simulink model "AIE_RTL_cosim_black_box"  (R2023a)
settings: Solver=VariableStepAuto  StartTime=0.0  StopTime=4000  RelTol=1e-3
PreLoadFcn:
  | xmcCheckSlxPath(bdroot);
  | input = readcomplexdata('./sw/input.h');
  | 
  | % ii of the HDL black box design is 19. Hence we are running
  | % the HDL desgin at 20 times faster than
  | % the input sample time.
  | 
  | sample_time = 0.5/20
InitFcn:
  | xlEvaluateHDLBlocks('AIE_RTL_cosim_black_box')
undefined symbols (not defined in the file): c, S, vsva2197, xcvc1902
libraries: hdlBasic x4, aieUtilities x2, aieBasic x2, hdlUtilities x2, simulink x1, dspsrcs4 x1, vmcUtilities x1
settings Model: Creator=abehbood  LastModifiedBy=robg
settings SolverCC: AlgebraicLoopSolver=TrustRegion
settings DebuggingCC: UnconnectedInputMsg=warning  UnconnectedOutputMsg=warning  UnconnectedLineMsg=warning
settings ModelReferenceCC: EnableRefExpFcnMdlSchedulingChecks=on
settings SFSimCC: CustomCodeUndefinedFunction=UseInterfaceOnly
settings RTWCC: DLArmComputeVersion=19.05

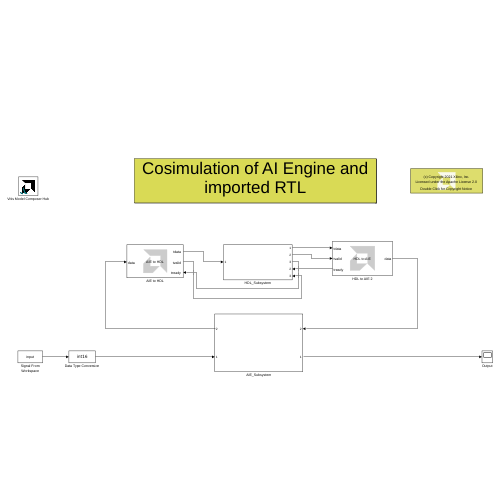
[thumbnail: Simulink's stored preview of the top-level diagram]
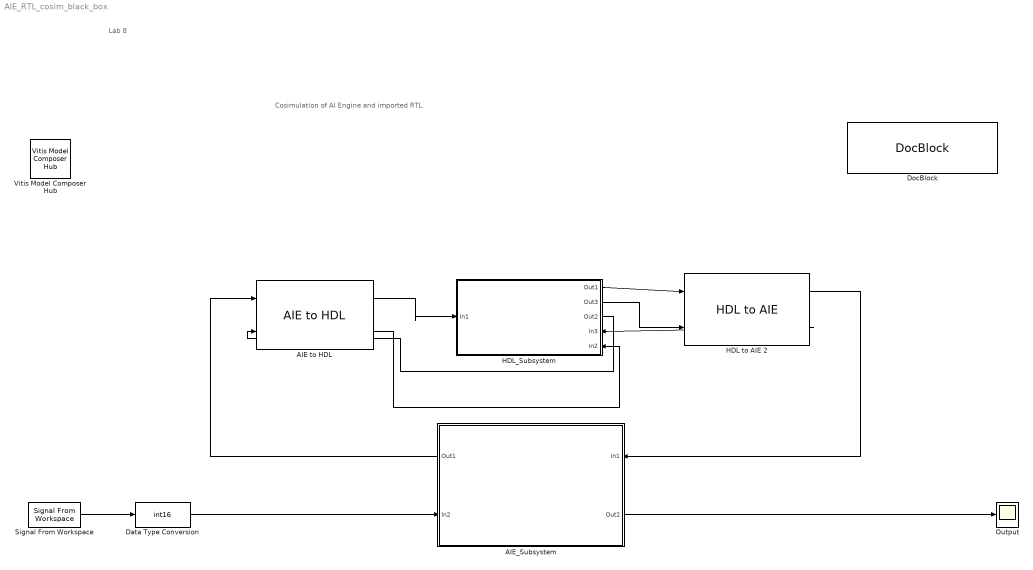
== system AIE_RTL_cosim_black_box ==
  note: Lab 8
  note: Cosimulation of AI Engine and imported RTL
  AIE to HDL : aieUtilities/AIE to HDL  OutDataType=uint32  OutSampleTime=Inherit: Same as tready
  AIE_Subsystem : Subsystem
      settings: PortSchema="{\"entries\":[{\"content\":{\"sides\":[{\"content\":{\"connectorIds\":[\"Out2\",\"In1\"]},\"type\":\"ConnectorPlacement.EquallySpacedRectSide\",\"uuid\":\"898d8c47-e932-4e65-b4ee-22fcab4c971c\"},{\"content\":{\"connectorIds\":[\"In2\",\"Out1\"],\"side\":\"RIGHT\"},\"type\":\"ConnectorPlacement.EquallySpacedRectSide\",\"uuid\":\"af23ae14-2da0-4d61-8b36-3a1d0e7ee3d3\"},{\"content\":{\"connectorIds\":[],\"side\":\"TOP\"},\"type\":\"ConnectorPlacement.EquallySpacedRectSide\",\"uuid\":\"f5229823-660d-4ed4-bac1-26d92dde4203\"}]},\"type\":\"ConnectorPlacement.EquallySpacedConnector\",\"uuid\":\"c8995052-e1b5-42bb-bdd0-b566c20174a5\"}],\"packageUris\":[\"http://schema.mathworks.com/mf0/Connector/19700101\"],\"version\":\"1.0\"}"
  Data Type Conversion : DataTypeConversion  OutDataTypeStr=int16  SaturateOnIntegerOverflow=off  RndMeth=Floor
  DocBlock : simulink/Model-Wide Utilities/DocBlock  DocumentType=Text  mask(DocBlock){}
      content=|
      | ///////////////////////////////////////////////////////////////////////////
      | // Copyright 2021 Xilinx
      | //
      | // Licensed under the Apache License, Version 2.0 (the "License");
      | // you may not use this file except in compliance with the License.
      | // You may obtain a copy of the License at
      | //
      | // http://www.apache.org/licenses/LICENSE-2.0
      | //
      | // Unless required by applicable law or agreed to in writing, software
      | // distributed under the License is distributed on an "AS IS" BASIS,
      | // WITHOUT WARRANTIES OR CONDITIONS OF ANY KIND, either express or implied.
      | // See the License for the specific language governing permissions and
      | // limitations under the License.
      | ///////////////////////////////////////////////////////////////////////////
      mask Display:
      | xmcDrawBlockIcon();
      | disp(['{\fontsize{10pt}(c) Copyright 2021' ' Xilinx, Inc.}\newline \newline '],'texmode','on');
      | disp('{\fontsize{10pt}Licensed under the Apache License 2.0}','texmode','on');
      | disp('\newline \newline \newline{\fontsize{10pt}Double Click for Copyright Notice}','texmode','on');
  HDL to AIE 2 : aieUtilities/HDL to AIE  InDataType=uint32  OutDataType=int16 (c)  OutSampleTime=.5  SamplesPerFrame=256  RateReduceFactor=1  ManuallySpecifyOutSampleTime=on
  HDL_Subsystem : Subsystem
      settings: PortSchema="{\"entries\":[{\"content\":{\"sides\":[{\"content\":{\"connectorIds\":[\"In1\"]},\"type\":\"ConnectorPlacement.EquallySpacedRectSide\",\"uuid\":\"f7d09b9b-9cab-45de-a234-ce17189f1f38\"},{\"content\":{\"connectorIds\":[\"Out1\",\"Out2\",\"Out3\",\"In2\",\"In3\"],\"side\":\"RIGHT\"},\"type\":\"ConnectorPlacement.EquallySpacedRectSide\",\"uuid\":\"963e2550-c982-4a72-83e5-f36d54b36baa\"},{\"content\":{\"connectorIds\":[],\"side\":\"TOP\"},\"type\":\"ConnectorPlacement.EquallySpacedRectSide\",\"uuid\":\"f90a1520-9218-4692-a090-e2089f523264\"}]},\"type\":\"ConnectorPlacement.EquallySpacedConnector\",\"uuid\":\"882f0c8e-c8d0-442e-9388-2de8afbb4cc9\"}],\"packageUris\":[\"http://schema.mathworks.com/mf0/Connector/R2020b\"],\"version\":\"1.0\"}"
  Output : Scope
  Signal From Workspace : dspsrcs4/Signal From Workspace  X=input  Ts=1  nsamps=128  OutputAfterFinalValue=Setting to zero  ignoreOrWarnInputAndFrameLengths=off  OutputFrames=off
  Vitis Model Composer Hub : vmcUtilities/Vitis Model Composer Hub  Tag=genX  CodeGeneration=off  SubsystemName=HDL_Subsystem  CompilationType=HDLCompilation  ExportTypeV2=IP Catalog  StartColumn=1  NumberOfColumns=1  TargetDirectory=./netlist/ip/HDL_Subsystem/src  exportDesign=off  analyzeDesign=on  validateDesignOnHw=off  ExportType=AI Engines  IpVendor=xilinx.com  IpLibrary=hls  IpVersion=1.0  IpHWLanguage=Verilog  AieCompilerOptions={}  AieSimulatorOptions={}  CreateTestbench=on  TestbenchStackSize=10  RunRtlSim=off  RunCSim=off  RunAieSim=off  AieSimTimeout=50000  RunAieSimProfiling=off  LaunchVitisAnalyzer=off  PlotOutput=off  RunX86Sim=off  X86SimTimeout=10  GenHwImage=off  GenLibadfXo=off  GenHwValidationCode=off  PlatformType=Not Specified  HwSystemType=Linux  HwValidationTarget=hw_emu  CommonSwDir=/proj/xbuilds/CustTA/2022.1_2022_0311_0103/internal_platforms/sw/versal/xilinx-versal-common-v2022.1  SdkDirectory=/proj/xsjhdstaff4/abehbood/petalinux/2022.1  ProjDevice=xcvc1902-vsva2197-1LP-e-S  ProjDevicePart=xcvc1902-vsva2197-1LP-e-S  AIEType=AIE  SamplePeriod=-1  ClockFrequency=200  DataPathParallelism=1  xilinxfamily=versalaicore  part=xcvc1902  speed=-1LP-e-S  package=vsva2197  directory=./netlist/ip/HDL_Subsystem/src  testbench=on  incr_netlist=off  synthesis_tool=Vivado  clock_wrapper=Clock Enables  dbl_ovrd=According to Block Masks  dcm_input_clock_period=10  sysclk_period=10  simulink_period=sample_time  eval_field=0  IPInfoJsonString="{\"HDLSubsystem\":{\"SubsystemName\":\"HDL_Subsystem\",\"IPName\":\"HDL_Subsystem\",\"IPLibrary\":\"VMC\",\"IPVendor\":\"User Company\",\"IPVersion\":\"1.0\",\"TargetDirectory\":\"./netlist\",\"SubsystemDir\":\"./netlist/ip/HDL_Subsystem\"},\"SubsystemTag\":\"HDLNode\"}"  LogFileName=''  NThreads=4
  wires:
  Signal From Workspace/1 -> Data Type Conversion/1
  HDL to AIE 2/1 -> AIE_Subsystem/2(In1)
  Data Type Conversion/1 -> AIE_Subsystem/1(In2)
  AIE_Subsystem/2(Out1) -> AIE to HDL/1
  AIE_Subsystem/1(Out2) -> Output/1
  AIE to HDL/1 -> HDL_Subsystem/1(In1)
  HDL to AIE 2/2 -> HDL_Subsystem/2(In3)
  HDL_Subsystem/1(Out1) -> HDL to AIE 2/1
  HDL_Subsystem/2(Out3) -> HDL to AIE 2/2
  HDL_Subsystem/3(Out2) -> AIE to HDL/2
  AIE to HDL/2 -> HDL_Subsystem/3(In2)

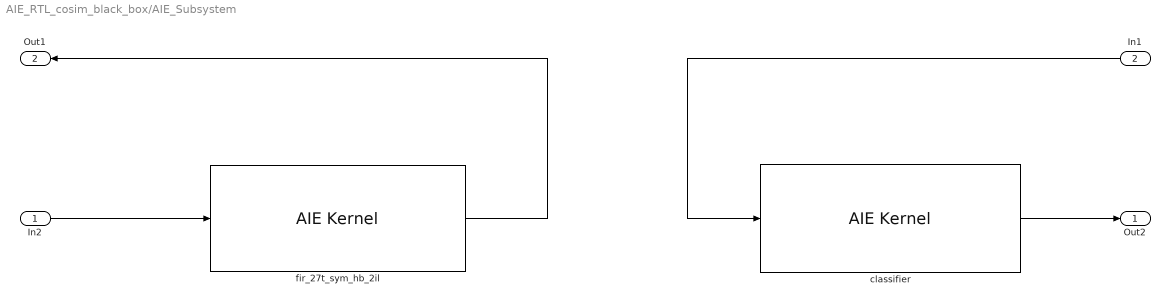
== system AIE_RTL_cosim_black_box/AIE_Subsystem ==
  In2 : Inport
  In1 : Inport  Port=2
  classifier : aieBasic/AIE Kernel  KernelAllAttrs=s[12;12;9;9;19;14;21;23;24;21;12;24;26;26;26;27;28;9;21;23;23;23;24;25;14;19;19;29]@FunctionNameDeclFileNamePortNamesPortTypesPortSerializedTypesPortDirectionsPortWindowSizeEnablesPortWindowMarginEnablesPortSynchronicityEnablesPortSignalSizeEnablesFunctionDeclFunctionTemplateSpecKindFunctionTemplateParamNamesFunctionTemplateParamKindsFunctionTemplateParamTypesFunctionTemplateParamValuesFunctionTemplateParamEnablesClassDeclClassTemplateSpecKindClassTemplateParamNamesClassTemplateParamKindsClassTemplateParamTypesClassTemplateParamValuesClassTemplateParamEnablesClassCtorDeclsClassCtorParamNamesClassCtorParamTypesClassCtorParamSerializedTypes[1 1]@C[28 1]@t10@classifiert19@../../src/kernels.hC[2 1]@t5@inputt6@outputC[2 1]@t21@input_stream_cint16 *t21@output_window_int32 *C[2 1]@t33@{P{Tinput_stream{1{t{Scint16}}}}}t31@{P{Toutput_window{1{t{Bi32}}}}}C[2 1]@t5@inputt6@outputC[2 1]@l0@l1@C[2 1]@l0@l0@C[2 1]@l0@l1@C[2 1]@l0@l0@t74@void classifier(input_stream_cint16 * input, output_window_int32 * output)t4@nonee[0 1]@e[0 1]@e[0 1]@e[0 1]@e[0 1]@nne[0 1]@e[0 1]@e[0 1]@e[0 1]@e[0 1]@e[0 1]@e[0 1]@e[0 1]@e[0 1]@  PortNames={'input'; 'output'}  PortSerializedTypes={'{P{Tinput_stream{1{t{Scint16}}}}}'; '{P{Toutput_window{1{t{Bi32}}}}}'}  PortWindowSizes={0.000000000000000000e+00, 2.560000000000000000e+02}  PortWindowMargins={0.000000000000000000e+00, 0.000000000000000000e+00}  PortSynchronicities={'auto', 'auto'}  PortSignalSizes={0.000000000000000000e+00; 0.000000000000000000e+00}  FunctionTemplateSpecKind=none  FunctionTemplateParamNames={}  FunctionTemplateParamKinds={}  FunctionTemplateParamTypes={}  FunctionTemplateParamValues={}  FunctionIndex=1  FunctionTabVisible=on  FunctionTemplateParamsVisible=off  FunctionDeclTypeOptions=C[1 1]@t74@void classifier(input_stream_cint16 * input, output_window_int32 * output)  FunctionDecl=void classifier(input_stream_cint16 * input, output_window_int32 * output)  FunctionTemplateParams={}  FunctionTemplateParamsEnables={}  PortAttrs={ 'Input', 'input', 'input_stream_cint16 *', '', '', '', ''; 'Output', 'output', 'output_window_int32 *', '256', '', 'auto', '' }  PortAttrsEnables={'off', 'off', 'off', 'off', 'off', 'off', 'off';'off', 'off', 'off', 'on', 'off', 'on', 'off'}  SampleTime=-1  KernelHeaderFile=src/kernels.h  KernelFunction=classifier  KernelSourceFile=src/kernels/classifiers/classify.cc  KernelSearchPaths={}  PreProcOptions={}  blockJsonConstraints=[]
  fir_27t_sym_hb_2il : aieBasic/AIE Kernel  KernelAllAttrs=s[12;12;9;9;19;14;21;23;24;21;12;24;26;26;26;27;28;9;21;23;23;23;24;25;14;19;19;29]@FunctionNameDeclFileNamePortNamesPortTypesPortSerializedTypesPortDirectionsPortWindowSizeEnablesPortWindowMarginEnablesPortSynchronicityEnablesPortSignalSizeEnablesFunctionDeclFunctionTemplateSpecKindFunctionTemplateParamNamesFunctionTemplateParamKindsFunctionTemplateParamTypesFunctionTemplateParamValuesFunctionTemplateParamEnablesClassDeclClassTemplateSpecKindClassTemplateParamNamesClassTemplateParamKindsClassTemplateParamTypesClassTemplateParamValuesClassTemplateParamEnablesClassCtorDeclsClassCtorParamNamesClassCtorParamTypesClassCtorParamSerializedTypes[1 1]@C[28 1]@t17@fir_27t_sym_hb_2it19@../../src/kernels.hC[2 1]@t7@inputcbt8@outputcbC[2 1]@t21@input_window_cint16 *t22@output_window_cint16 *C[2 1]@t33@{P{Tinput_window{1{t{Scint16}}}}}t34@{P{Toutput_window{1{t{Scint16}}}}}C[2 1]@t5@inputt6@outputC[2 1]@l1@l1@C[2 1]@l1@l0@C[2 1]@l1@l1@C[2 1]@l0@l0@t86@void fir_27t_sym_hb_2i(input_window_cint16 * inputcb, output_window_cint16 * outputcb)t4@nonee[0 1]@e[0 1]@e[0 1]@e[0 1]@e[0 1]@nne[0 1]@e[0 1]@e[0 1]@e[0 1]@e[0 1]@e[0 1]@e[0 1]@e[0 1]@e[0 1]@  PortNames={'inputcb'; 'outputcb'}  PortSerializedTypes={'{P{Tinput_window{1{t{Scint16}}}}}'; '{P{Toutput_window{1{t{Scint16}}}}}'}  PortWindowSizes={1.280000000000000000e+02, 2.560000000000000000e+02}  PortWindowMargins={1.600000000000000000e+01, 0.000000000000000000e+00}  PortSynchronicities={'auto', 'auto'}  PortSignalSizes={0.000000000000000000e+00; 0.000000000000000000e+00}  FunctionTemplateSpecKind=none  FunctionTemplateParamNames={}  FunctionTemplateParamKinds={}  FunctionTemplateParamTypes={}  FunctionTemplateParamValues={}  FunctionIndex=1  FunctionTabVisible=on  FunctionTemplateParamsVisible=off  FunctionDeclTypeOptions=C[1 1]@t86@void fir_27t_sym_hb_2i(input_window_cint16 * inputcb, output_window_cint16 * outputcb)  FunctionDecl=void fir_27t_sym_hb_2i(input_window_cint16 * inputcb, output_window_cint16 * outputcb)  FunctionTemplateParams={}  FunctionTemplateParamsEnables={}  PortAttrs={ 'Input','inputcb','input_window_cint16 *','128','16','auto','';'Output','outputcb','output_window_cint16 *','256','','auto','' }  PortAttrsEnables={'off', 'off', 'off', 'on', 'on', 'on', 'off';'off', 'off', 'off', 'on', 'off', 'on', 'off'}  SampleTime=-1  KernelHeaderFile=src/kernels.h  KernelFunction=fir_27t_sym_hb_2i  KernelSourceFile=src/kernels/interpolators/hb27_2i.cc  KernelSearchPaths={}  PreProcOptions={}  blockJsonConstraints=[]
  Out2 : Outport
  Out1 : Outport  Port=2
  wires:
  classifier/1 -> Out2/1
  In2/1 -> fir_27t_sym_hb_2il/1
  In1/1 -> classifier/1
  fir_27t_sym_hb_2il/1 -> Out1/1

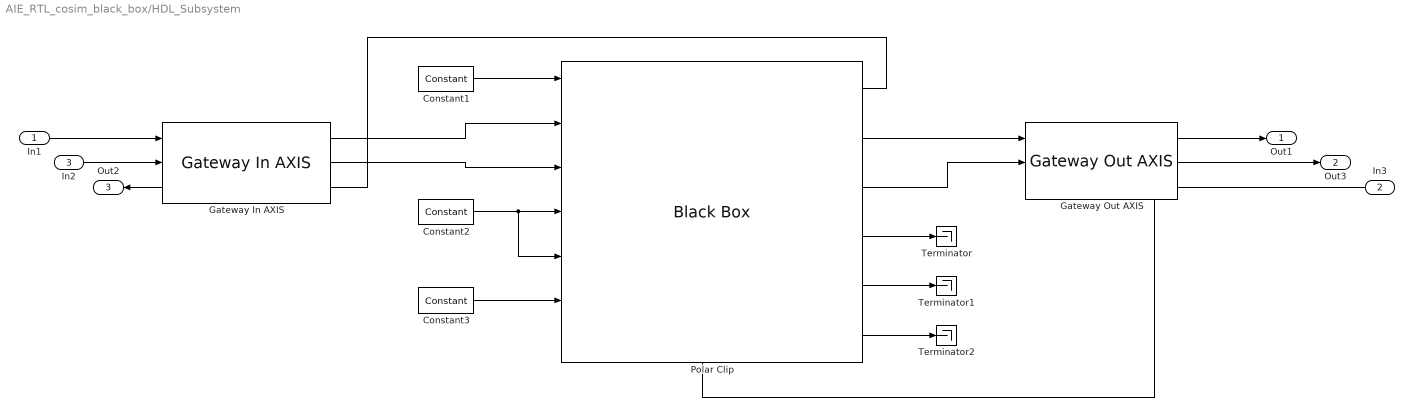
== system AIE_RTL_cosim_black_box/HDL_Subsystem ==
  In1 : Inport
  In3 : Inport  Port=2
  In2 : Inport  Port=3
  Constant1 : hdlBasic/Constant  const=1  gui_display_data_type=Boolean  arith_type=Boolean  n_bits=16  bin_pt=14  preci_type=Single  exp_width=8  frac_width=24  explicit_period=on  period=sample_time  XmcBlockStatus=1  maskContainerNames=tabcontainer1  block_type=constant  block_config=sysgen:Constant_config
  Constant2 : hdlBasic/Constant  const=15  gui_display_data_type=Fixed-point  arith_type=Unsigned  n_bits=4  bin_pt=0  preci_type=Single  exp_width=8  frac_width=24  explicit_period=on  period=sample_time  XmcBlockStatus=1  maskContainerNames=tabcontainer1  block_type=constant  block_config=sysgen:Constant_config
  Constant3 : hdlBasic/Constant  const=0  gui_display_data_type=Boolean  arith_type=Boolean  n_bits=16  bin_pt=14  preci_type=Single  exp_width=8  frac_width=24  explicit_period=on  period=sample_time  XmcBlockStatus=1  maskContainerNames=tabcontainer1  block_type=constant  block_config=sysgen:Constant_config
  Gateway In AXIS : hdlUtilities/Gateway In AXIS  gui_display_data_type=Fixed-point  arith_type=Unsigned  n_bits=32  bin_pt=0  preci_type=Custom  exp_width=16  frac_width=24  quantization="Round  (unbiased: +/- Inf)"  overflow=Saturate  OutSampleTime=sample_time  block_type=gatewayinaxi  XmcBlockStatus=1
  Gateway Out AXIS : hdlUtilities/Gateway Out AXIS  mask_sample_period=sample_time  block_type=gatewayoutaxi
  Polar Clip : hdlBasic/Black Box  init_code=polar_clip_config  sim_method=Vivado Simulator  verbose=off  XmcBlockStatus=1  maskContainerNames=group1  block_type=blackbox2  block_config=sysgen:black_box_config
  Terminator : Terminator
  Terminator1 : Terminator
  Terminator2 : Terminator
  Out1 : Outport
  Out3 : Outport  Port=2
  Out2 : Outport  Port=3
  wires:
  Constant2/1 -> Polar Clip/5, Polar Clip/4
  Polar Clip/4 -> Terminator/1
  Polar Clip/6 -> Terminator2/1
  Polar Clip/5 -> Terminator1/1
  Constant1/1 -> Polar Clip/1
  Polar Clip/1 -> Gateway In AXIS/3
  Constant3/1 -> Polar Clip/6
  Polar Clip/3 -> Gateway Out AXIS/2
  Gateway Out AXIS/2 -> Out3/1
  Gateway In AXIS/2 -> Polar Clip/3
  Gateway In AXIS/1 -> Polar Clip/2
  Gateway In AXIS/3 -> Out2/1
  In1/1 -> Gateway In AXIS/1
  In2/1 -> Gateway In AXIS/2
  Polar Clip/2 -> Gateway Out AXIS/1
  Gateway Out AXIS/1 -> Out1/1
  In3/1 -> Gateway Out AXIS/3
  Gateway Out AXIS/3 -> Polar Clip/7
